simulink model "zad1"  (R2025a)
settings: Solver=VariableStepAuto  StartTime=0.0  StopTime=3500  RelTol=1e-3
libraries: fuzblock x3
settings Model: Creator=jovan  LastModifiedBy=jovan

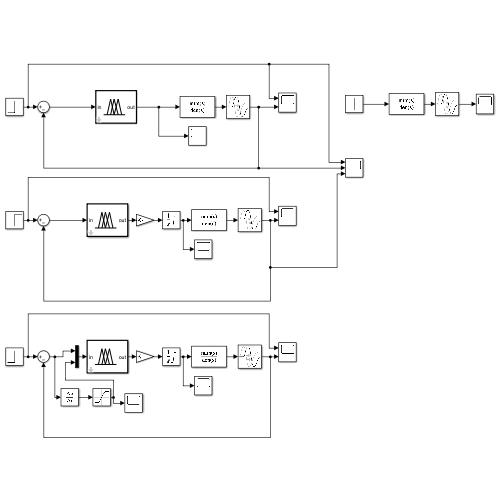
[thumbnail: Simulink's stored preview of the top-level diagram]
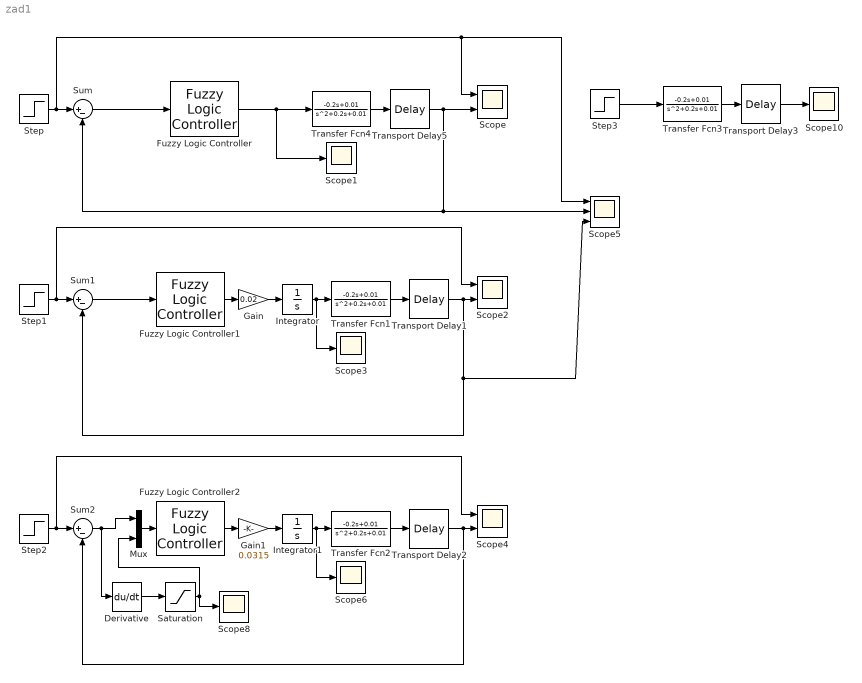
== system zad1 ==
  Derivative : Derivative
  Fuzzy Logic Controller : fuzblock/Fuzzy Logic  Controller  FIS='fuzzyZadatakA1.fis'  OutputSampleNumber=101  DataType=double  UseLookupTable=off  NumBreakpoints=10  FuzzifiedInputs=off  RuleFiringStrengths=off  RuleOutputs=off  AggregatedOutputs=off  SimulateUsing=Interpreted execution  OutOfRangeInputValueMessage=warning  NoRuleFiredMessage=warning  EmptyOutputFuzzySetMessage=warning
  Fuzzy Logic Controller1 : fuzblock/Fuzzy Logic  Controller  FIS='fuzzyZadatakA1.fis'  OutputSampleNumber=101  DataType=double  UseLookupTable=off  NumBreakpoints=10  FuzzifiedInputs=off  RuleFiringStrengths=off  RuleOutputs=off  AggregatedOutputs=off  SimulateUsing=Interpreted execution  OutOfRangeInputValueMessage=warning  NoRuleFiredMessage=warning  EmptyOutputFuzzySetMessage=warning
  Fuzzy Logic Controller2 : fuzblock/Fuzzy Logic  Controller  FIS='fuzzyZadatakA.fis'  OutputSampleNumber=101  DataType=double  UseLookupTable=off  NumBreakpoints=10  FuzzifiedInputs=off  RuleFiringStrengths=off  RuleOutputs=off  AggregatedOutputs=off  SimulateUsing=Interpreted execution  OutOfRangeInputValueMessage=warning  NoRuleFiredMessage=warning  EmptyOutputFuzzySetMessage=warning
  Gain : Gain  Gain=0.02
  Gain1 : Gain  Gain=0.0315
  Integrator : Integrator  LimitOutput=on  UpperSaturationLimit=1.5  LowerSaturationLimit=-1.5
  Integrator1 : Integrator  LimitOutput=on  UpperSaturationLimit=1.5  LowerSaturationLimit=-1.5
  Mux : Mux  Inputs=2
  Saturation : Saturate  UpperLimit=0.1  LowerLimit=-0.1
  Scope : Scope  NumInputPorts=2
      settings: ActiveDisplayYMinimum=-1  ActiveDisplayYMaximum=1
  Scope{1,3,6,8,10} (5 alike) : Scope
      Scope1 settings: ActiveDisplayYMinimum=-1  ActiveDisplayYMaximum=1
      Scope10 settings: ActiveDisplayYMinimum=-1  ActiveDisplayYMaximum=1  DataLoggingVariableName=ScopeData7
      Scope3 settings: ActiveDisplayYMinimum=-1  ActiveDisplayYMaximum=1  DataLoggingVariableName=ScopeData3
      Scope6 settings: ActiveDisplayYMinimum=-1  ActiveDisplayYMaximum=1  DataLoggingVariableName=ScopeData6
      Scope8 settings: ActiveDisplayYMinimum=-1  ActiveDisplayYMaximum=1  DataLoggingVariableName=ScopeData9
  Scope2 : Scope  NumInputPorts=2
      settings: ActiveDisplayYMinimum=-2.90611251206115  ActiveDisplayYMaximum=0.9162161886124579  DataLoggingVariableName=ScopeData2
  Scope4 : Scope  NumInputPorts=2
      settings: ActiveDisplayYMinimum=-2.90611251206115  ActiveDisplayYMaximum=0.9162161886124579  DataLoggingVariableName=ScopeData4
  Scope5 : Scope  NumInputPorts=3
      settings: ActiveDisplayYMinimum=-1  ActiveDisplayYMaximum=1  DataLoggingVariableName=ScopeData5
  Step{,1..3} (4 alike) : Step  Time=1100  Before=-1  SampleTime=0
  Sum : Sum  Inputs=|+-
  Sum1 : Sum  Inputs=|+-
  Sum2 : Sum  Inputs=|+-
  Transfer Fcn{1..4} (4 alike) : TransferFcn  Numerator=[-0.2 0.01]  Denominator=[1 0.2 0.01]
  Transport Delay{1..3,5} (4 alike) : TransportDelay  DelayTime=4
  wires:
  Transfer Fcn4/1 -> Transport Delay5/1
  Fuzzy Logic Controller/1 -> Transfer Fcn4/1, Scope1/1
  Sum/1 -> Fuzzy Logic Controller/1
  Transport Delay5/1 -> Scope/2, Scope5/2, Sum/2
  Step1/1 -> Sum1/1, Scope2/1
  Step/1 -> Scope5/1, Scope/1, Sum/1
  Transfer Fcn1/1 -> Transport Delay1/1
  Transport Delay1/1 -> Sum1/2, Scope5/3, Scope2/2
  Step3/1 -> Transfer Fcn3/1
  Transfer Fcn3/1 -> Transport Delay3/1
  Transport Delay3/1 -> Scope10/1
  Integrator/1 -> Scope3/1, Transfer Fcn1/1
  Fuzzy Logic Controller1/1 -> Gain/1
  Gain/1 -> Integrator/1
  Transfer Fcn2/1 -> Transport Delay2/1
  Fuzzy Logic Controller2/1 -> Gain1/1
  Step2/1 -> Scope4/1, Sum2/1
  Integrator1/1 -> Scope6/1, Transfer Fcn2/1
  Transport Delay2/1 -> Scope4/2, Sum2/2
  Gain1/1 -> Integrator1/1
  Mux/1 -> Fuzzy Logic Controller2/1
  Sum2/1 -> Mux/1, Derivative/1
  Derivative/1 -> Saturation/1
  Saturation/1 -> Scope8/1, Mux/2
  Sum1/1 -> Fuzzy Logic Controller1/1
